simulink model "ExtendedSimulink"  (Simulink 7.1)
settings: Solver=FixedStepDiscrete  StartTime=0.0  StopTime=inf  RelTol=1e-3  SampleTimeConstraint=Specified
PreLoadFcn:
  | setpaths
InitFcn:
  | clear;
  | home;
  | disp('Starting FAMOUSO ...')
  | global input_channel_IDs;
  | global output_channel_IDs;
StartFcn:
  | FAMOUSOconnectAll();
  | FAMOUSOsubscribeAll();
  | FAMOUSOannounceAll();
StopFcn:
  | FAMOUSOdisconnectAll();
  | disp('Aus Maus')
undefined symbols (not defined in the file or in its folder): get_events, Simulink_get_data, Simulink_publish
settings Model: Creator=Sebastian Zug  LastModifiedBy=zug
settings MATStruct: SampleTime=0.05  Offset=0  Priority=[10.0]

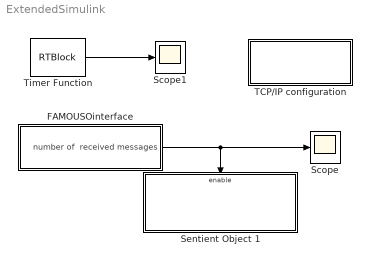
== system ExtendedSimulink ==
  FAMOUSOinterface : Subsystem
  Scope : Scope
      settings: YMin=0  YMax=2
  Scope1 : Scope
      settings: YMin=0  YMax=50  SaveName=timing  DataFormat=Array
  Sentient Object 1 : Subsystem
      mask Display: image(imread('figures/SentientObject.jpg'))
  TCP/IP configuration : Subsystem  Priority=1  mask(COSMIC TCP/IP Configuration){IP='127.0.0.1', Port=5005}
      mask init:
      | disp('Configuration of the network connection')
      | global TCPIPsettings;
      | 
      | TCPIPsettings.host=strrep(get_param(gcb, 'IP'), '''', '');
      | TCPIPsettings.port=str2num(get_param(gcb, 'Port'));
      mask Display: fprintf('%s\n %s',get_param(gcb, 'IP'),get_param(gcb, 'Port'))
  Timer Function : S-Function  FunctionName=RTBlock  Parameters=step,TaskPriority,ThPriority  EnableBusSupport=off  mask(RTBlock){step=50, TaskPriority=HIGH, ThPriority=TIME CRITICAL}
      mask prompts: step "Timestep (ms)"; TaskPriority "Task Priority"; ThPriority "Thread Priority"
      mask help:
      | Real Time Block: Set the characteristics of a real-time simulation. The settings of the simulation are selectable using the block panel. The parameters are:
      |
      | - Timeout: in milliseconds, defines the temporization with which Simulink requires to the Operating System the availability of resources for the execution of the simulation step. The value should be fixed equal to the simulation step of Simulink (the timestep);
      |
      | - Priority Class: defines the class of task priority required, that can be one of the following values:
      | -- IDLE PRIORITY: Low priority, typical of an idle process (priority less than normal)
      | -- NORMAL PRIORITY: Typical priority of a typical windows application;
      | -- HIGH PRIORITY: Typical priority of a relevant application, that needs more resources of a normal application;
      | -- REAL-TIME PRIORITY: Exclusive priority of a unique process that needs all the resources of the operating system.
      |
      | - Thread Priority: defines the class of task priority required, that can be one of the following values:
      | -- IDLE : The thread should run when the main process is inactive.
      | -- LOWEST : The thread runs with a minimal respect of the temporization;
      | -- NORMAL : The thread runs with the same priority of the main process;
      | -- HIGH : The thread runs with the major priority respect to the main process;
      | -- REAL-TIME : The process runs when the simulation thread is in idle state.
      mask StyleString: edit,popup(IDLE|NORMAL|HIGH|REAL-TIME),popup(IDLE|LOWEST|NORMAL|HIGHEST|TIME CRITICAL)
  wires:
  FAMOUSOinterface/1(number of  received messages) -> Scope/1, Sentient Object 1/Enable
  Timer Function/1 -> Scope1/1

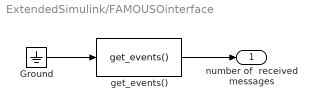
== system ExtendedSimulink/FAMOUSOinterface ==
  Ground : Ground
  get_events() : MATLABFcn  MATLABFcn=get_events()  OutputSignalType=real  Output1D=off
  number of  received messages : Outport  OutDataType=sfix(16)  OutScaling=2^0
  wires:
  get_events()/1 -> number of  received messages/1
  Ground/1 -> get_events()/1

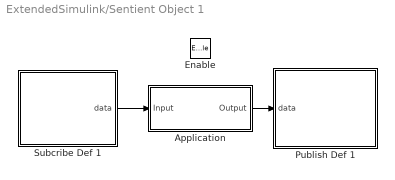
== system ExtendedSimulink/Sentient Object 1 ==
  Enable : EnablePort
  Application : Subsystem
  Publish Def 1 : Subsystem  mask(COSMIC Publish Channel){subject='F300000000000000', subject_dec=17509995351216488000, nickname='distance'}
      mask prompts: subject_dec "Subject decimal"; nickname "Name"
      mask help: This Box defines the COSMIC Channels for Output
      mask init:
      | clear global output_channel_IDs
      | global output_channel_IDs
      | 
      | subject=strrep(get_param(gcb, 'subject'), '''', '');
      | comment=strrep(get_param(gcb, 'nickname'), '''', '');
      | aux=0;
      | value=deblank(subject);
      | for i=1:8
      |      aux=aux+hex2dec(value(2*i-1:2*i))*256^(8-i); 
      | end
      | set_param(gcb, 'subject_dec',num2str(aux));
      | 
      | 
      | exists_already=0;
      | % if isempty(output_channel_IDs)
      | %     output_channel_IDs=struct('name',{},'subject',{});  
      | %     fprintf('\n           subject            comment\n-----------------------------------------------\n');
      |      i=1;
      | % else
      | %     for j=1:size(output_channel_IDs,2)
      | %         if strcmp(output_channel_IDs(j).subject,subject)
      | %             exists_already=1;
      | %             break;
      | %         else
      | %             if strcmp(output_channel_IDs(j).name,comment)
      | %                 error('same nicknames used !!!')
      | %             end
      | %         end
      | %     end
      | % end
      | % if ~exists_already
      | %     i=size(output_channel_IDs,2)+1;
      |     %Ausgabe auf der Konsole
      | %     fprintf('publish    %s   %s\n', subject, comment);
      |     % Anlegen der globalen Variablen
      |     eval(sprintf('global %s;',comment));
      |     %Initialisieren
      |     eval(sprintf('%s=output_channel(subject, comment);', comment));
      | 	output_channel_IDs(i).name=comment;
      | 	output_channel_IDs(i).subject=subject;
      |     
      | % end
      | 
      | global TCPIPsettings;
      | 
      | aux=TCPIP_connection();
      |     aux=set_properties(aux,'host',TCPIPsettings.host);
      |     aux=set_properties(aux,'port',TCPIPsettings.port);
      |     for i=1:get_output_channel_info('size')
      |         channel_name=get_output_channel_info('channel_name',i);
      |         eval(sprintf('global %s;',channel_name));
      |         aux=set_properties(aux,'interaction_type','polling');
      |         eval(sprintf('%s=set_properties(%s,''connection'',aux);',char(channel_name),char(channel_name)));
      |     end
      settings: AttributesFormatString=%<subject>\n%<nickname>
      mask Help:
      | The form allows 4 parameter:
      | * Subject - a 64 Byte Identifier
      | * Name
      mask CallbackString:
      | if size(get_param(gcb, 'subject'))~=[1 16]
      |    disp('Bitte einen 64 Byte hexdezimalen Wert eingeben')
      | end||
      mask Display:
      | fprintf('Publish \n%s\n %s',get_param(gcb, 'subject'),get_param(gcb, 'nickname'))
      | image(imread('figures/SentientObjectOutput.jpg'))
  Subcribe Def 1 : Subsystem  mask(COSMIC Subscribed Channel){subject='F200000000000000', subject_dec=17437937757178561000, nickname='robot', number=0, timeout=0}
      mask prompts: subject_dec "Subject dec"; nickname "Name"
      mask help: This Box defines the COSMIC Channels for Input
      mask init:
      | clear global input_channel_IDs;
      | global input_channel_IDs
      | 
      | subject=strrep(get_param(gcb, 'subject'), '''', '');
      | subject=char(subject);
      | comment=strrep(get_param(gcb, 'nickname'), '''', '');
      | timeout=1;
      | number=8;
      | aux=0;
      | value=deblank(subject);
      | for i=1:8
      |      aux=aux+hex2dec(value(2*i-1:2*i))*256^(8-i); 
      | end
      | set_param(gcb, 'subject_dec',num2str(aux));
      | 
      | exists_already=0;
      | %if isempty(input_channel_IDs)
      | %     input_channel_IDs=struct('name',{},'subject',{});  
      | %     fprintf('\n           subject            comment\n-----------------------------------------------\n');
      |     i=1;
      | % else
      | %     for j=1:size(input_channel_IDs,2)
      | %         if strcmp(input_channel_IDs(j).subject,subject)
      | %             exists_already=1;
      | %             break;
      | %         else
      | %             if strcmp(input_channel_IDs(j).name,comment)
      | %                 error('same nicknames used !!!')
      | %             end
      | %         end
      | %     end
      | % end
      | %if ~exists_already
      |    % i=size(input_channel_IDs,2)+1;
      |     %Ausgabe auf der Konsole
      | %     fprintf('subscribe  %s   %s\n', subject, comment);
      |     % Anlegen der globalen Variablen
      |     eval(sprintf('global %s;',comment));
      |     %Initialisieren
      |     %eval(sprintf('%s=input_channel(subject, timeout, number, comment);', comment));
      |     eval(sprintf('%s=input_channel(char(subject), number, char(comment), ''-'');',char(comment)));
      | 	input_channel_IDs(i).name=comment;
      | 	input_channel_IDs(i).subject=subject;
      | %end
      | 
      | 
      | global TCPIPsettings;
      | 
      | if get_input_channel_info('size')>0
      |     aux=TCPIP_connection();
      |     aux=set_properties(aux,'host',TCPIPsettings.host);
      |     aux=set_properties(aux,'port',TCPIPsettings.port);
      |     aux=set_properties(aux,'message_length',21); 
      |     for i=1:get_input_channel_info('size')
      |         channel_name=get_input_channel_info('channel_name',i);
      |         aux=set_properties(aux,'channel_name',channel_name);
      |         eval(sprintf('global %s;',channel_name));
      |         aux=set_properties(aux,'interaction_type','polling');     
      |         eval(sprintf('%s=set_properties(%s,''connection'',aux);',char(channel_name),char(channel_name)));
      |     end
      | end
      settings: AttributesFormatString=%<subject>\n%<nickname>
      mask Help:
      | The form allows 4 parameter:
      | * Subject - a 64 Byte Identifier
      | * Name
      | * Number
      | * Size
      mask CallbackString:
      | if size(get_param(gcb, 'subject'))~=[1 16]
      |    disp('Bitte einen 64 Byte hexdezimalen Wert eingeben')
      | end||||
      mask Display:
      | fprintf('Subcribe\n%s\n %s',get_param(gcb, 'subject'),get_param(gcb, 'nickname'))
      | image(imread('figures/SentientObjectInput.jpg'));
  wires:
  Subcribe Def 1/1(data) -> Application/1(Input)
  Application/1(Output) -> Publish Def 1/1(data)

== system ExtendedSimulink/TCP/IP configuration ==

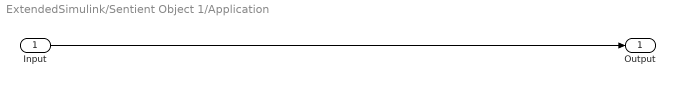
== system ExtendedSimulink/Sentient Object 1/Application ==
  Input : Inport  PortDimensions=[1 8]  OutDataType=sfix(16)  OutScaling=2^0
  Output : Outport  OutDataType=sfix(16)  OutScaling=2^0
  wires:
  Input/1 -> Output/1

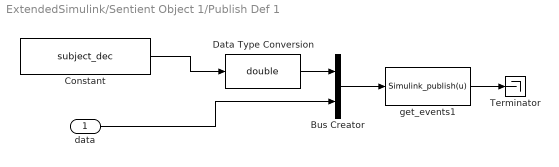
== system ExtendedSimulink/Sentient Object 1/Publish Def 1 ==
  data : Inport  PortDimensions=[1 8]  OutDataType=sfix(16)  OutScaling=2^0
  Bus Creator : BusCreator  Inputs=2
  Constant : Constant  Value=subject_dec  OutDataType=sfix(16)  OutScaling=2^0
  Data Type Conversion : DataTypeConversion  OutDataTypeMode=double  OutDataType=fixdt(0,64)  OutDataTypeStr=double  RndMeth=Zero
  Terminator : Terminator
  get_events1 : MATLABFcn  MATLABFcn=Simulink_publish(u)  OutputDimensions=[1 1]  OutputSignalType=real  Output1D=off
  wires:
  Bus Creator/1 -> get_events1/1
  get_events1/1 -> Terminator/1
  data/1 -> Bus Creator/2
  Data Type Conversion/1 -> Bus Creator/1
  Constant/1 -> Data Type Conversion/1

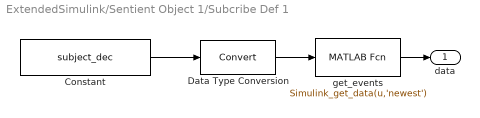
== system ExtendedSimulink/Sentient Object 1/Subcribe Def 1 ==
  Constant : Constant  Value=subject_dec  OutDataType=sfix(16)  OutScaling=2^0
  Data Type Conversion : DataTypeConversion  OutDataType=sfix(16)  OutScaling=2^0
  get_events : MATLABFcn  MATLABFcn=Simulink_get_data(u,'newest')  OutputSignalType=real  Output1D=off
  data : Outport  OutDataType=sfix(16)  OutScaling=2^0
  wires:
  Constant/1 -> Data Type Conversion/1
  Data Type Conversion/1 -> get_events/1
  get_events/1 -> data/1
